simulink library "AtomicLibrary"
PostLoadFcn:
  | PacketBusGenerator
libraries: LinkLayer x5

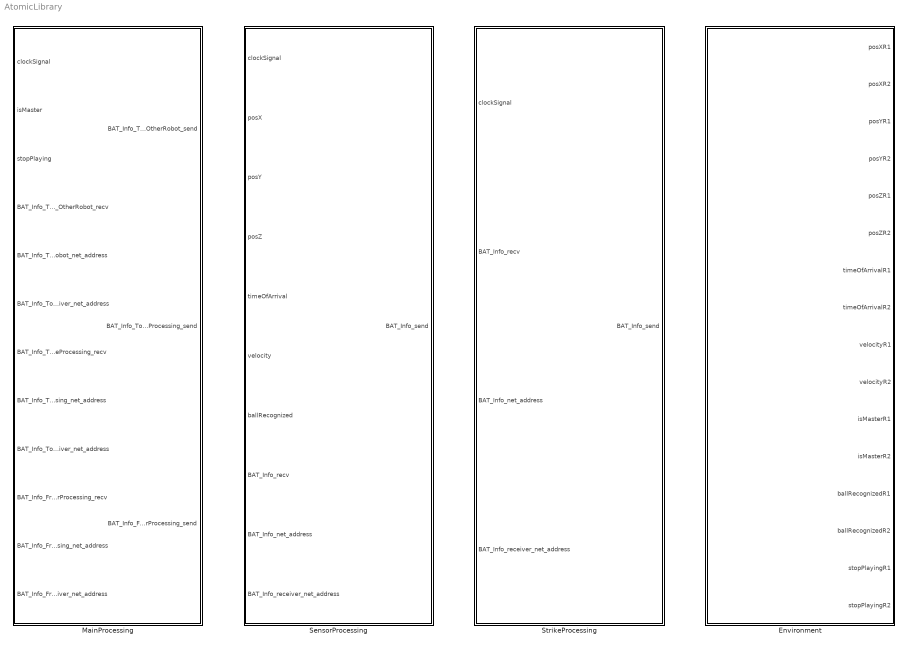
== system AtomicLibrary ==
  MainProcessing : Subsystem  Tag=id=_SXgnIKYDEeKR7Lwk7UC7tQ
  SensorProcessing : Subsystem  Tag=id=_SYKHYKYDEeKR7Lwk7UC7tQ
  StrikeProcessing : Subsystem  Tag=id=_SYeQcKYDEeKR7Lwk7UC7tQ
  Environment : Subsystem  Tag=id=_SY2q8KYDEeKR7Lwk7UC7tQ

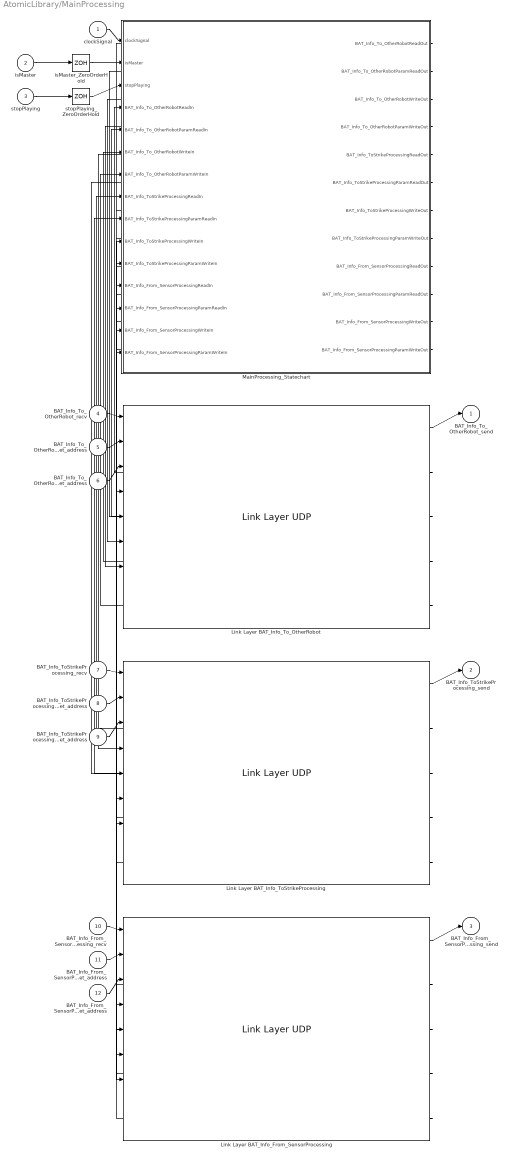
== system AtomicLibrary/MainProcessing ==
  clockSignal : Inport  Tag=id=_SXupkKYDEeKR7Lwk7UC7tQ  Port=1  DataType=auto  OutDataType=fixdt(1, 16)  OutScaling=2^0  OutDataTypeStr=Inherit: auto
  isMaster : Inport  Tag=id=_SmZ-wKYDEeKR7Lwk7UC7tQ  Port=2  DataType=boolean  OutDataType=fixdt(1, 16)  OutScaling=2^0  OutDataTypeStr=boolean
  stopPlaying : Inport  Tag=id=_SnFUMKYDEeKR7Lwk7UC7tQ  Port=3  DataType=boolean  OutDataType=fixdt(1, 16)  OutScaling=2^0  OutDataTypeStr=boolean
  BAT_Info_To_OtherRobot_recv : Inport  Tag=id=_StHDsKYDEeKR7Lwk7UC7tQ  Port=4  DataType=auto  OutDataType=fixdt(1, 16)  OutScaling=2^0  UseBusObject=on  OutDataTypeStr=Inherit: auto
      settings: BusObject=PacketBus
  BAT_Info_To_OtherRobot_net_address : Inport  Tag=id=_StIR0aYDEeKR7Lwk7UC7tQ  Port=5  DataType=uint8  OutDataType=fixdt(1, 16)  OutScaling=2^0  OutDataTypeStr=uint8
  BAT_Info_To_OtherRobot_receiver_net_address : Inport  Tag=id=_StI44KYDEeKR7Lwk7UC7tQ  Port=6  DataType=uint8  OutDataType=fixdt(1, 16)  OutScaling=2^0  OutDataTypeStr=uint8
  BAT_Info_ToStrikeProcessing_recv : Inport  Tag=id=_St01YKYDEeKR7Lwk7UC7tQ  Port=7  DataType=auto  OutDataType=fixdt(1, 16)  OutScaling=2^0  UseBusObject=on  OutDataTypeStr=Inherit: auto
      settings: BusObject=PacketBus
  BAT_Info_ToStrikeProcessing_net_address : Inport  Tag=id=_St3RoKYDEeKR7Lwk7UC7tQ  Port=8  DataType=uint8  OutDataType=fixdt(1, 16)  OutScaling=2^0  OutDataTypeStr=uint8
  BAT_Info_ToStrikeProcessing_receiver_net_address : Inport  Tag=id=_St34sKYDEeKR7Lwk7UC7tQ  Port=9  DataType=uint8  OutDataType=fixdt(1, 16)  OutScaling=2^0  OutDataTypeStr=uint8
  BAT_Info_From_SensorProcessing_recv : Inport  Tag=id=_SujOIKYDEeKR7Lwk7UC7tQ  Port=10  DataType=auto  OutDataType=fixdt(1, 16)  OutScaling=2^0  UseBusObject=on  OutDataTypeStr=Inherit: auto
      settings: BusObject=PacketBus
  BAT_Info_From_SensorProcessing_net_address : Inport  Tag=id=_SulqYKYDEeKR7Lwk7UC7tQ  Port=11  DataType=uint8  OutDataType=fixdt(1, 16)  OutScaling=2^0  OutDataTypeStr=uint8
  BAT_Info_From_SensorProcessing_receiver_net_address : Inport  Tag=id=_SunfkKYDEeKR7Lwk7UC7tQ  Port=12  DataType=uint8  OutDataType=fixdt(1, 16)  OutScaling=2^0  OutDataTypeStr=uint8
  BAT_Info_To_OtherRobot_send : Outport  Tag=id=_StGcoKYDEeKR7Lwk7UC7tQ  Port=1  DataType=auto  OutDataType=fixdt(1, 16)  OutScaling=2^0  UseBusObject=on  OutDataTypeStr=Inherit: auto
      settings: BusObject=PacketBus
  BAT_Info_ToStrikeProcessing_send : Outport  Tag=id=_St0OUKYDEeKR7Lwk7UC7tQ  Port=2  DataType=auto  OutDataType=fixdt(1, 16)  OutScaling=2^0  UseBusObject=on  OutDataTypeStr=Inherit: auto
      settings: BusObject=PacketBus
  BAT_Info_From_SensorProcessing_send : Outport  Tag=id=_SuinEKYDEeKR7Lwk7UC7tQ  Port=3  DataType=auto  OutDataType=fixdt(1, 16)  OutScaling=2^0  UseBusObject=on  OutDataTypeStr=Inherit: auto
      settings: BusObject=PacketBus
  MainProcessing_Statechart : Stateflow chart  Tag=id=_SXeK4KYDEeKR7Lwk7UC7tQ
  isMaster_ZeroOrderHold : ZeroOrderHold  Tag=id=_Smk94KYDEeKR7Lwk7UC7tQ  SampleTime=10.0
  stopPlaying_ZeroOrderHold : ZeroOrderHold  Tag=id=_SnJloKYDEeKR7Lwk7UC7tQ  SampleTime=10.0
  Link Layer BAT_Info_To_OtherRobot : LinkLayer/Link Layer UDP  DelayMin=2  DelayMax=100  MessageLossProbability=0
  Link Layer BAT_Info_ToStrikeProcessing : LinkLayer/Link Layer UDP  DelayMin=2  DelayMax=100  MessageLossProbability=0
  Link Layer BAT_Info_From_SensorProcessing : LinkLayer/Link Layer UDP  DelayMin=2  DelayMax=100  MessageLossProbability=0
  wires:
  clockSignal/1 -> MainProcessing_Statechart/1(clockSignal)
  isMaster/1 -> isMaster_ZeroOrderHold/1
  isMaster_ZeroOrderHold/1 -> MainProcessing_Statechart/2(isMaster)
  stopPlaying/1 -> stopPlaying_ZeroOrderHold/1
  stopPlaying_ZeroOrderHold/1 -> MainProcessing_Statechart/3(stopPlaying)
  Link Layer BAT_Info_To_OtherRobot/1 -> BAT_Info_To_OtherRobot_send/1
  BAT_Info_To_OtherRobot_recv/1 -> Link Layer BAT_Info_To_OtherRobot/1
  MainProcessing_Statechart/1(BAT_Info_To_OtherRobotReadOut) -> Link Layer BAT_Info_To_OtherRobot/4
  Link Layer BAT_Info_To_OtherRobot/2 -> MainProcessing_Statechart/4(BAT_Info_To_OtherRobotReadIn)
  Link Layer BAT_Info_To_OtherRobot/3 -> MainProcessing_Statechart/5(BAT_Info_To_OtherRobotParamReadIn)
  MainProcessing_Statechart/2(BAT_Info_To_OtherRobotParamReadOut) -> Link Layer BAT_Info_To_OtherRobot/5
  MainProcessing_Statechart/3(BAT_Info_To_OtherRobotWriteOut) -> Link Layer BAT_Info_To_OtherRobot/6
  MainProcessing_Statechart/4(BAT_Info_To_OtherRobotParamWriteOut) -> Link Layer BAT_Info_To_OtherRobot/7
  Link Layer BAT_Info_To_OtherRobot/4 -> MainProcessing_Statechart/6(BAT_Info_To_OtherRobotWriteIn)
  Link Layer BAT_Info_To_OtherRobot/5 -> MainProcessing_Statechart/7(BAT_Info_To_OtherRobotParamWriteIn)
  BAT_Info_To_OtherRobot_net_address/1 -> Link Layer BAT_Info_To_OtherRobot/2
  BAT_Info_To_OtherRobot_receiver_net_address/1 -> Link Layer BAT_Info_To_OtherRobot/3
  Link Layer BAT_Info_ToStrikeProcessing/1 -> BAT_Info_ToStrikeProcessing_send/1
  BAT_Info_ToStrikeProcessing_recv/1 -> Link Layer BAT_Info_ToStrikeProcessing/1
  MainProcessing_Statechart/5(BAT_Info_ToStrikeProcessingReadOut) -> Link Layer BAT_Info_ToStrikeProcessing/4
  Link Layer BAT_Info_ToStrikeProcessing/2 -> MainProcessing_Statechart/8(BAT_Info_ToStrikeProcessingReadIn)
  Link Layer BAT_Info_ToStrikeProcessing/3 -> MainProcessing_Statechart/9(BAT_Info_ToStrikeProcessingParamReadIn)
  MainProcessing_Statechart/6(BAT_Info_ToStrikeProcessingParamReadOut) -> Link Layer BAT_Info_ToStrikeProcessing/5
  MainProcessing_Statechart/7(BAT_Info_ToStrikeProcessingWriteOut) -> Link Layer BAT_Info_ToStrikeProcessing/6
  MainProcessing_Statechart/8(BAT_Info_ToStrikeProcessingParamWriteOut) -> Link Layer BAT_Info_ToStrikeProcessing/7
  Link Layer BAT_Info_ToStrikeProcessing/4 -> MainProcessing_Statechart/10(BAT_Info_ToStrikeProcessingWriteIn)
  Link Layer BAT_Info_ToStrikeProcessing/5 -> MainProcessing_Statechart/11(BAT_Info_ToStrikeProcessingParamWriteIn)
  BAT_Info_ToStrikeProcessing_net_address/1 -> Link Layer BAT_Info_ToStrikeProcessing/2
  BAT_Info_ToStrikeProcessing_receiver_net_address/1 -> Link Layer BAT_Info_ToStrikeProcessing/3
  Link Layer BAT_Info_From_SensorProcessing/1 -> BAT_Info_From_SensorProcessing_send/1
  BAT_Info_From_SensorProcessing_recv/1 -> Link Layer BAT_Info_From_SensorProcessing/1
  MainProcessing_Statechart/9(BAT_Info_From_SensorProcessingReadOut) -> Link Layer BAT_Info_From_SensorProcessing/4
  Link Layer BAT_Info_From_SensorProcessing/2 -> MainProcessing_Statechart/12(BAT_Info_From_SensorProcessingReadIn)
  Link Layer BAT_Info_From_SensorProcessing/3 -> MainProcessing_Statechart/13(BAT_Info_From_SensorProcessingParamReadIn)
  MainProcessing_Statechart/10(BAT_Info_From_SensorProcessingParamReadOut) -> Link Layer BAT_Info_From_SensorProcessing/5
  MainProcessing_Statechart/11(BAT_Info_From_SensorProcessingWriteOut) -> Link Layer BAT_Info_From_SensorProcessing/6
  MainProcessing_Statechart/12(BAT_Info_From_SensorProcessingParamWriteOut) -> Link Layer BAT_Info_From_SensorProcessing/7
  Link Layer BAT_Info_From_SensorProcessing/4 -> MainProcessing_Statechart/14(BAT_Info_From_SensorProcessingWriteIn)
  Link Layer BAT_Info_From_SensorProcessing/5 -> MainProcessing_Statechart/15(BAT_Info_From_SensorProcessingParamWriteIn)
  BAT_Info_From_SensorProcessing_net_address/1 -> Link Layer BAT_Info_From_SensorProcessing/2
  BAT_Info_From_SensorProcessing_receiver_net_address/1 -> Link Layer BAT_Info_From_SensorProcessing/3

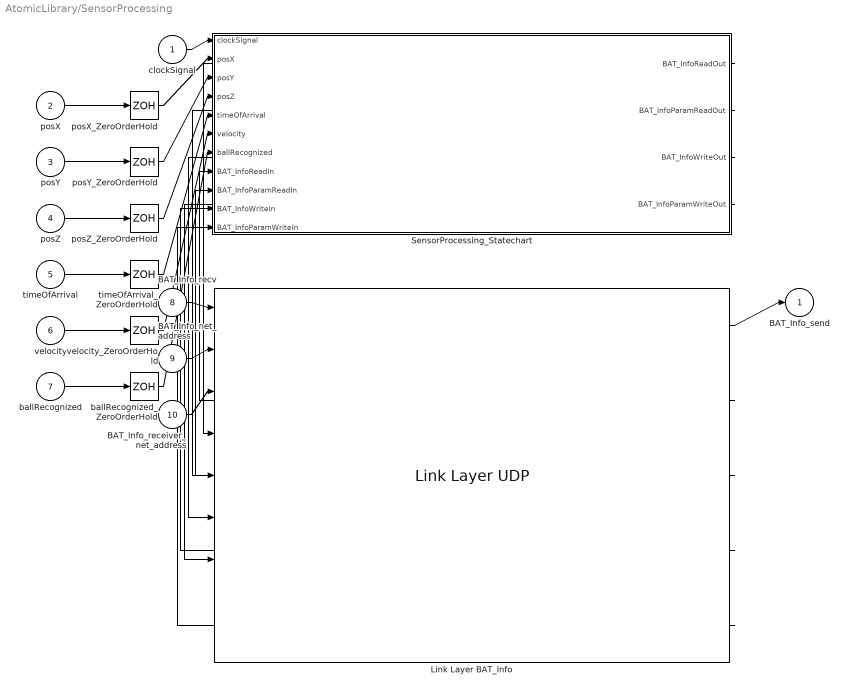
== system AtomicLibrary/SensorProcessing ==
  clockSignal : Inport  Tag=id=_SYLVgKYDEeKR7Lwk7UC7tQ  Port=1  DataType=auto  OutDataType=fixdt(1, 16)  OutScaling=2^0  OutDataTypeStr=Inherit: auto
  posX : Inport  Tag=id=_SnjOQKYDEeKR7Lwk7UC7tQ  Port=2  DataType=double  OutDataType=fixdt(1, 16)  OutScaling=2^0  OutDataTypeStr=double
  posY : Inport  Tag=id=_SoH2AKYDEeKR7Lwk7UC7tQ  Port=3  DataType=double  OutDataType=fixdt(1, 16)  OutScaling=2^0  OutDataTypeStr=double
  posZ : Inport  Tag=id=_SoozYKYDEeKR7Lwk7UC7tQ  Port=4  DataType=double  OutDataType=fixdt(1, 16)  OutScaling=2^0  OutDataTypeStr=double
  timeOfArrival : Inport  Tag=id=_SpS6sKYDEeKR7Lwk7UC7tQ  Port=5  DataType=double  OutDataType=fixdt(1, 16)  OutScaling=2^0  OutDataTypeStr=double
  velocity : Inport  Tag=id=_Sp5XoKYDEeKR7Lwk7UC7tQ  Port=6  DataType=double  OutDataType=fixdt(1, 16)  OutScaling=2^0  OutDataTypeStr=double
  ballRecognized : Inport  Tag=id=_SqplkKYDEeKR7Lwk7UC7tQ  Port=7  DataType=boolean  OutDataType=fixdt(1, 16)  OutScaling=2^0  OutDataTypeStr=boolean
  BAT_Info_recv : Inport  Tag=id=_SvNVcKYDEeKR7Lwk7UC7tQ  Port=8  DataType=auto  OutDataType=fixdt(1, 16)  OutScaling=2^0  UseBusObject=on  OutDataTypeStr=Inherit: auto
      settings: BusObject=PacketBus
  BAT_Info_net_address : Inport  Tag=id=_SvPKoKYDEeKR7Lwk7UC7tQ  Port=9  DataType=uint8  OutDataType=fixdt(1, 16)  OutScaling=2^0  OutDataTypeStr=uint8
  BAT_Info_receiver_net_address : Inport  Tag=id=_SvPxsKYDEeKR7Lwk7UC7tQ  Port=10  DataType=uint8  OutDataType=fixdt(1, 16)  OutScaling=2^0  OutDataTypeStr=uint8
  BAT_Info_send : Outport  Tag=id=_SvMuYKYDEeKR7Lwk7UC7tQ  Port=1  DataType=auto  OutDataType=fixdt(1, 16)  OutScaling=2^0  UseBusObject=on  OutDataTypeStr=Inherit: auto
      settings: BusObject=PacketBus
  SensorProcessing_Statechart : Stateflow chart  Tag=id=_SYI5QKYDEeKR7Lwk7UC7tQ
  posX_ZeroOrderHold : ZeroOrderHold  Tag=id=_Snm4oKYDEeKR7Lwk7UC7tQ  SampleTime=10.0
  posY_ZeroOrderHold : ZeroOrderHold  Tag=id=_SoK5UKYDEeKR7Lwk7UC7tQ  SampleTime=10.0
  posZ_ZeroOrderHold : ZeroOrderHold  Tag=id=_Sotr4KYDEeKR7Lwk7UC7tQ  SampleTime=10.0
  timeOfArrival_ZeroOrderHold : ZeroOrderHold  Tag=id=_SpXMIKYDEeKR7Lwk7UC7tQ  SampleTime=10.0
  velocity_ZeroOrderHold : ZeroOrderHold  Tag=id=_Sp_eQKYDEeKR7Lwk7UC7tQ  SampleTime=10.0
  ballRecognized_ZeroOrderHold : ZeroOrderHold  Tag=id=_SqtP8KYDEeKR7Lwk7UC7tQ  SampleTime=10.0
  Link Layer BAT_Info : LinkLayer/Link Layer UDP  DelayMin=2  DelayMax=100  MessageLossProbability=0
  wires:
  clockSignal/1 -> SensorProcessing_Statechart/1(clockSignal)
  posX/1 -> posX_ZeroOrderHold/1
  posX_ZeroOrderHold/1 -> SensorProcessing_Statechart/2(posX)
  posY/1 -> posY_ZeroOrderHold/1
  posY_ZeroOrderHold/1 -> SensorProcessing_Statechart/3(posY)
  posZ/1 -> posZ_ZeroOrderHold/1
  posZ_ZeroOrderHold/1 -> SensorProcessing_Statechart/4(posZ)
  timeOfArrival/1 -> timeOfArrival_ZeroOrderHold/1
  timeOfArrival_ZeroOrderHold/1 -> SensorProcessing_Statechart/5(timeOfArrival)
  velocity/1 -> velocity_ZeroOrderHold/1
  velocity_ZeroOrderHold/1 -> SensorProcessing_Statechart/6(velocity)
  ballRecognized/1 -> ballRecognized_ZeroOrderHold/1
  ballRecognized_ZeroOrderHold/1 -> SensorProcessing_Statechart/7(ballRecognized)
  Link Layer BAT_Info/1 -> BAT_Info_send/1
  BAT_Info_recv/1 -> Link Layer BAT_Info/1
  SensorProcessing_Statechart/1(BAT_InfoReadOut) -> Link Layer BAT_Info/4
  Link Layer BAT_Info/2 -> SensorProcessing_Statechart/8(BAT_InfoReadIn)
  Link Layer BAT_Info/3 -> SensorProcessing_Statechart/9(BAT_InfoParamReadIn)
  SensorProcessing_Statechart/2(BAT_InfoParamReadOut) -> Link Layer BAT_Info/5
  SensorProcessing_Statechart/3(BAT_InfoWriteOut) -> Link Layer BAT_Info/6
  SensorProcessing_Statechart/4(BAT_InfoParamWriteOut) -> Link Layer BAT_Info/7
  Link Layer BAT_Info/4 -> SensorProcessing_Statechart/10(BAT_InfoWriteIn)
  Link Layer BAT_Info/5 -> SensorProcessing_Statechart/11(BAT_InfoParamWriteIn)
  BAT_Info_net_address/1 -> Link Layer BAT_Info/2
  BAT_Info_receiver_net_address/1 -> Link Layer BAT_Info/3

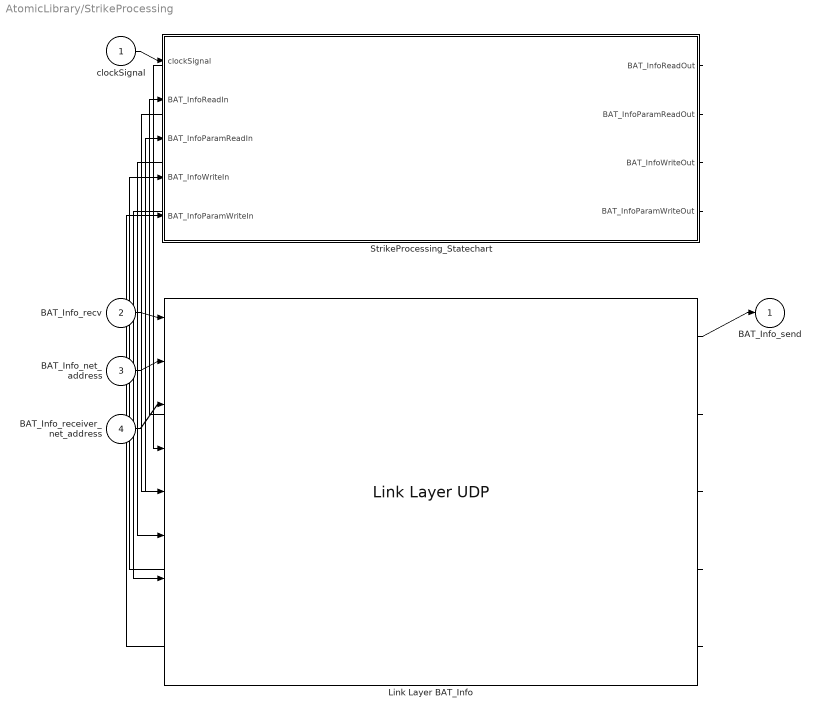
== system AtomicLibrary/StrikeProcessing ==
  clockSignal : Inport  Tag=id=_SYgFoKYDEeKR7Lwk7UC7tQ  Port=1  DataType=auto  OutDataType=fixdt(1, 16)  OutScaling=2^0  OutDataTypeStr=Inherit: auto
  BAT_Info_recv : Inport  Tag=id=_SsIMQKYDEeKR7Lwk7UC7tQ  Port=2  DataType=auto  OutDataType=fixdt(1, 16)  OutScaling=2^0  UseBusObject=on  OutDataTypeStr=Inherit: auto
      settings: BusObject=PacketBus
  BAT_Info_net_address : Inport  Tag=id=_SsYD4KYDEeKR7Lwk7UC7tQ  Port=3  DataType=uint8  OutDataType=fixdt(1, 16)  OutScaling=2^0  OutDataTypeStr=uint8
  BAT_Info_receiver_net_address : Inport  Tag=id=_SsZSAKYDEeKR7Lwk7UC7tQ  Port=4  DataType=uint8  OutDataType=fixdt(1, 16)  OutScaling=2^0  OutDataTypeStr=uint8
  BAT_Info_send : Outport  Tag=id=_SsG-IKYDEeKR7Lwk7UC7tQ  Port=1  DataType=auto  OutDataType=fixdt(1, 16)  OutScaling=2^0  UseBusObject=on  OutDataTypeStr=Inherit: auto
      settings: BusObject=PacketBus
  StrikeProcessing_Statechart : Stateflow chart  Tag=id=_SYbNIKYDEeKR7Lwk7UC7tQ
  Link Layer BAT_Info : LinkLayer/Link Layer UDP  DelayMin=2  DelayMax=100  MessageLossProbability=0
  wires:
  clockSignal/1 -> StrikeProcessing_Statechart/1(clockSignal)
  Link Layer BAT_Info/1 -> BAT_Info_send/1
  BAT_Info_recv/1 -> Link Layer BAT_Info/1
  StrikeProcessing_Statechart/1(BAT_InfoReadOut) -> Link Layer BAT_Info/4
  Link Layer BAT_Info/2 -> StrikeProcessing_Statechart/2(BAT_InfoReadIn)
  Link Layer BAT_Info/3 -> StrikeProcessing_Statechart/3(BAT_InfoParamReadIn)
  StrikeProcessing_Statechart/2(BAT_InfoParamReadOut) -> Link Layer BAT_Info/5
  StrikeProcessing_Statechart/3(BAT_InfoWriteOut) -> Link Layer BAT_Info/6
  StrikeProcessing_Statechart/4(BAT_InfoParamWriteOut) -> Link Layer BAT_Info/7
  Link Layer BAT_Info/4 -> StrikeProcessing_Statechart/4(BAT_InfoWriteIn)
  Link Layer BAT_Info/5 -> StrikeProcessing_Statechart/5(BAT_InfoParamWriteIn)
  BAT_Info_net_address/1 -> Link Layer BAT_Info/2
  BAT_Info_receiver_net_address/1 -> Link Layer BAT_Info/3

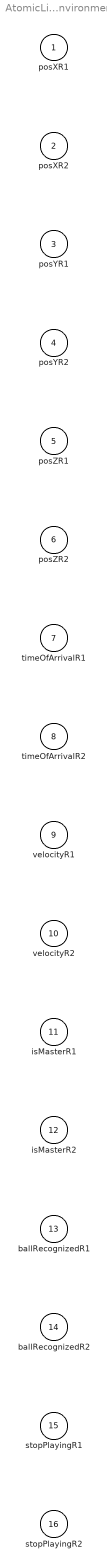
== system AtomicLibrary/Environment ==
  posXR1 : Outport  Tag=id=_SfmMIKYDEeKR7Lwk7UC7tQ  Port=1  DataType=double  OutDataType=fixdt(1, 16)  OutScaling=2^0  OutDataTypeStr=double
  posXR2 : Outport  Tag=id=_SgUk4KYDEeKR7Lwk7UC7tQ  Port=2  DataType=double  OutDataType=fixdt(1, 16)  OutScaling=2^0  OutDataTypeStr=double
  posYR1 : Outport  Tag=id=_Sg3-gKYDEeKR7Lwk7UC7tQ  Port=3  DataType=double  OutDataType=fixdt(1, 16)  OutScaling=2^0  OutDataTypeStr=double
  posYR2 : Outport  Tag=id=_Shr20KYDEeKR7Lwk7UC7tQ  Port=4  DataType=double  OutDataType=fixdt(1, 16)  OutScaling=2^0  OutDataTypeStr=double
  posZR1 : Outport  Tag=id=_Sh-xwKYDEeKR7Lwk7UC7tQ  Port=5  DataType=double  OutDataType=fixdt(1, 16)  OutScaling=2^0  OutDataTypeStr=double
  posZR2 : Outport  Tag=id=_SiMNIKYDEeKR7Lwk7UC7tQ  Port=6  DataType=double  OutDataType=fixdt(1, 16)  OutScaling=2^0  OutDataTypeStr=double
  timeOfArrivalR1 : Outport  Tag=id=_Sia2oKYDEeKR7Lwk7UC7tQ  Port=7  DataType=double  OutDataType=fixdt(1, 16)  OutScaling=2^0  OutDataTypeStr=double
  timeOfArrivalR2 : Outport  Tag=id=_SitKgKYDEeKR7Lwk7UC7tQ  Port=8  DataType=double  OutDataType=fixdt(1, 16)  OutScaling=2^0  OutDataTypeStr=double
  velocityR1 : Outport  Tag=id=_SjBTkKYDEeKR7Lwk7UC7tQ  Port=9  DataType=double  OutDataType=fixdt(1, 16)  OutScaling=2^0  OutDataTypeStr=double
  velocityR2 : Outport  Tag=id=_SjP9EKYDEeKR7Lwk7UC7tQ  Port=10  DataType=double  OutDataType=fixdt(1, 16)  OutScaling=2^0  OutDataTypeStr=double
  isMasterR1 : Outport  Tag=id=_SjgbwKYDEeKR7Lwk7UC7tQ  Port=11  DataType=boolean  OutDataType=fixdt(1, 16)  OutScaling=2^0  OutDataTypeStr=boolean
  isMasterR2 : Outport  Tag=id=_SjtQEKYDEeKR7Lwk7UC7tQ  Port=12  DataType=boolean  OutDataType=fixdt(1, 16)  OutScaling=2^0  OutDataTypeStr=boolean
  ballRecognizedR1 : Outport  Tag=id=_Sj-84KYDEeKR7Lwk7UC7tQ  Port=13  DataType=boolean  OutDataType=fixdt(1, 16)  OutScaling=2^0  OutDataTypeStr=boolean
  ballRecognizedR2 : Outport  Tag=id=_SkRQwKYDEeKR7Lwk7UC7tQ  Port=14  DataType=boolean  OutDataType=fixdt(1, 16)  OutScaling=2^0  OutDataTypeStr=boolean
  stopPlayingR1 : Outport  Tag=id=_Sky1MKYDEeKR7Lwk7UC7tQ  Port=15  DataType=boolean  OutDataType=fixdt(1, 16)  OutScaling=2^0  OutDataTypeStr=boolean
  stopPlayingR2 : Outport  Tag=id=_SlXc8KYDEeKR7Lwk7UC7tQ  Port=16  DataType=boolean  OutDataType=fixdt(1, 16)  OutScaling=2^0  OutDataTypeStr=boolean

== stateflow chart MainProcessing/MainProcessing_Statechart ==
  state chart
    state chartRegion [parallel]
      settings: executionOrder=2
      state init
        state MainProcessingPort_BAT_Info_To_Other_Robot [parallel]
          settings: executionOrder=3
          state Init
          state YourTurn
            entry: c0=reset();
          state MyTurn
            entry: c0=reset();
          state Timeout
          state Inv_Error
          Init -> YourTurn [order 2] : [isMaster == true && BAT_Info_ReceivedBySP == true]
              | {[BAT_Info_To_OtherRobotWriteOut, BAT_Info_To_OtherRobotParamWriteOut] = BAT_Info_To_OtherRobot_enqueue(EVT_TURN_POSX, BAT_Info_To_OtherRobotWriteOut, double(posXReceivedBySP), BAT_Info_To_OtherRobotParamWriteOut)
              | [BAT_Info_To_OtherRobotWriteOut, BAT_Info_To_OtherRobotParamWriteOut] = BAT_Info_To_OtherRobot_enqueue(EVT_TURN_POSY, BAT_Info_To_OtherRobotWriteOut, double(posYReceivedBySP), BAT_Info_To_OtherRobotParamWriteOut)
              | [BAT_Info_To_OtherRobotWriteOut, BAT_Info_To_OtherRobotParamWriteOut] = BAT_Info_To_OtherRobot_enqueue(EVT_TURN_POSZ, BAT_Info_To_OtherRobotWriteOut, double(posZReceivedBySP), BAT_Info_To_OtherRobotParamWriteOut)
              | [BAT_Info_To_OtherRobotWriteOut, BAT_Info_To_OtherRobotParamWriteOut] = BAT_Info_To_OtherRobot_enqueue(EVT_TURN_TIMEOFARRIVAL, BAT_Info_To_OtherRobotWriteOut, double(timeOfArrivalReceivedBySP), BAT_Info_To_OtherRobotParamWriteOut)
              | [BAT_Info_To_OtherRobotWriteOut, BAT_Info_To_OtherRobotParamWriteOut] = BAT_Info_To_OtherRobot_enqueue(EVT_TURN_VELOCITY, BAT_Info_To_OtherRobotWriteOut, double(velocityReceivedBySP), BAT_Info_To_OtherRobotParamWriteOut)
              | ; BAT_Info_ReceivedBySP = false ; }
          YourTurn -> Init [order 1] : [BAT_Info_To_OtherRobot_checkQueue(EVT_STOPPLAYING, BAT_Info_To_OtherRobotReadOut)]
              | {[BAT_Info_To_OtherRobotReadOut, BAT_Info_To_OtherRobotParamReadOut] = BAT_Info_To_OtherRobot_dequeue(EVT_STOPPLAYING, BAT_Info_To_OtherRobotReadOut, BAT_Info_To_OtherRobotParamReadOut); }
          MyTurn -> Init [order 1] : [stopPlaying == true]
              | {[BAT_Info_To_OtherRobotWriteOut, BAT_Info_To_OtherRobotParamWriteOut] = BAT_Info_To_OtherRobot_enqueue(EVT_STOPPLAYING, BAT_Info_To_OtherRobotWriteOut, 0, BAT_Info_To_OtherRobotParamWriteOut); }
          Timeout -> Init
          Init -> MyTurn [order 1] : [BAT_Info_To_OtherRobot_checkQueue(EVT_TURN_POSX, BAT_Info_To_OtherRobotReadOut) && BAT_Info_To_OtherRobot_checkQueue(EVT_TURN_POSY, BAT_Info_To_OtherRobotReadOut) && BAT_Info_To_OtherRobot_checkQueue(EVT_TURN_POSZ, BAT_Info_To_OtherRobotReadOut) && BAT_Info_To_OtherRobot_checkQueue(EVT_TURN_TIMEOFARRIVAL, BAT_Info_To_OtherRobotReadOut) && BAT_Info_To_OtherRobot_checkQueue(EVT_TURN_VELOCITY, BAT_Info_To_OtherRobotReadOut)]
              | {[BAT_Info_To_OtherRobotReadOut, BAT_Info_To_OtherRobotParamReadOut, tmp_var_1] = BAT_Info_To_OtherRobot_dequeue(EVT_TURN_POSX, BAT_Info_To_OtherRobotReadOut, BAT_Info_To_OtherRobotParamReadOut);
              | [BAT_Info_To_OtherRobotReadOut, BAT_Info_To_OtherRobotParamReadOut, tmp_var_2] = BAT_Info_To_OtherRobot_dequeue(EVT_TURN_POSY, BAT_Info_To_OtherRobotReadOut, BAT_Info_To_OtherRobotParamReadOut);
              | [BAT_Info_To_OtherRobotReadOut, BAT_Info_To_OtherRobotParamReadOut, tmp_var_3] = BAT_Info_To_OtherRobot_dequeue(EVT_TURN_POSZ, BAT_Info_To_OtherRobotReadOut, BAT_Info_To_OtherRobotParamReadOut);
              | [BAT_Info_To_OtherRobotReadOut, BAT_Info_To_OtherRobotParamReadOut, tmp_var_4] = BAT_Info_To_OtherRobot_dequeue(EVT_TURN_TIMEOFARRIVAL, BAT_Info_To_OtherRobotReadOut, BAT_Info_To_OtherRobotParamReadOut);
              | [BAT_Info_To_OtherRobotReadOut, BAT_Info_To_OtherRobotParamReadOut, tmp_var_5] = BAT_Info_To_OtherRobot_dequeue(EVT_TURN_VELOCITY, BAT_Info_To_OtherRobotReadOut, BAT_Info_To_OtherRobotParamReadOut); posXReceivedByRobot = tmp_var_1 ;  posYReceivedByRobot = tmp_var_2 ;  posZReceivedByRobot = tmp_var_3 ;  timeOfArrivalReceivedByRobot = tmp_var_4 ;  velocityReceivedByRobot = tmp_var_5 ;  BAT_Info_ReceivedByRobot = true ; }
          MyTurn -> YourTurn [order 3] : [BAT_Info_ReceivedBySP == true]
              | {[BAT_Info_To_OtherRobotWriteOut, BAT_Info_To_OtherRobotParamWriteOut] = BAT_Info_To_OtherRobot_enqueue(EVT_TURN_POSX, BAT_Info_To_OtherRobotWriteOut, double(posXReceivedByRobot), BAT_Info_To_OtherRobotParamWriteOut)
              | [BAT_Info_To_OtherRobotWriteOut, BAT_Info_To_OtherRobotParamWriteOut] = BAT_Info_To_OtherRobot_enqueue(EVT_TURN_POSY, BAT_Info_To_OtherRobotWriteOut, double(posYReceivedBySP), BAT_Info_To_OtherRobotParamWriteOut)
              | [BAT_Info_To_OtherRobotWriteOut, BAT_Info_To_OtherRobotParamWriteOut] = BAT_Info_To_OtherRobot_enqueue(EVT_TURN_POSZ, BAT_Info_To_OtherRobotWriteOut, double(posZReceivedBySP), BAT_Info_To_OtherRobotParamWriteOut)
              | [BAT_Info_To_OtherRobotWriteOut, BAT_Info_To_OtherRobotParamWriteOut] = BAT_Info_To_OtherRobot_enqueue(EVT_TURN_TIMEOFARRIVAL, BAT_Info_To_OtherRobotWriteOut, double(timeOfArrivalReceivedBySP), BAT_Info_To_OtherRobotParamWriteOut)
              | [BAT_Info_To_OtherRobotWriteOut, BAT_Info_To_OtherRobotParamWriteOut] = BAT_Info_To_OtherRobot_enqueue(EVT_TURN_VELOCITY, BAT_Info_To_OtherRobotWriteOut, double(velocityReceivedBySP), BAT_Info_To_OtherRobotParamWriteOut)
              | ; BAT_Info_ReceivedBySP = false ; }
          YourTurn -> MyTurn [order 3] : [BAT_Info_To_OtherRobot_checkQueue(EVT_TURN_POSX, BAT_Info_To_OtherRobotReadOut) && BAT_Info_To_OtherRobot_checkQueue(EVT_TURN_POSY, BAT_Info_To_OtherRobotReadOut) && BAT_Info_To_OtherRobot_checkQueue(EVT_TURN_POSZ, BAT_Info_To_OtherRobotReadOut) && BAT_Info_To_OtherRobot_checkQueue(EVT_TURN_TIMEOFARRIVAL, BAT_Info_To_OtherRobotReadOut) && BAT_Info_To_OtherRobot_checkQueue(EVT_TURN_VELOCITY, BAT_Info_To_OtherRobotReadOut)]
              | {[BAT_Info_To_OtherRobotReadOut, BAT_Info_To_OtherRobotParamReadOut, tmp_var_1] = BAT_Info_To_OtherRobot_dequeue(EVT_TURN_POSX, BAT_Info_To_OtherRobotReadOut, BAT_Info_To_OtherRobotParamReadOut);
              | [BAT_Info_To_OtherRobotReadOut, BAT_Info_To_OtherRobotParamReadOut, tmp_var_2] = BAT_Info_To_OtherRobot_dequeue(EVT_TURN_POSY, BAT_Info_To_OtherRobotReadOut, BAT_Info_To_OtherRobotParamReadOut);
              | [BAT_Info_To_OtherRobotReadOut, BAT_Info_To_OtherRobotParamReadOut, tmp_var_3] = BAT_Info_To_OtherRobot_dequeue(EVT_TURN_POSZ, BAT_Info_To_OtherRobotReadOut, BAT_Info_To_OtherRobotParamReadOut);
              | [BAT_Info_To_OtherRobotReadOut, BAT_Info_To_OtherRobotParamReadOut, tmp_var_4] = BAT_Info_To_OtherRobot_dequeue(EVT_TURN_TIMEOFARRIVAL, BAT_Info_To_OtherRobotReadOut, BAT_Info_To_OtherRobotParamReadOut);
              | [BAT_Info_To_OtherRobotReadOut, BAT_Info_To_OtherRobotParamReadOut, tmp_var_5] = BAT_Info_To_OtherRobot_dequeue(EVT_TURN_VELOCITY, BAT_Info_To_OtherRobotReadOut, BAT_Info_To_OtherRobotParamReadOut); posXReceivedByRobot = tmp_var_1 ;  posYReceivedByRobot = tmp_var_2 ;  posZReceivedByRobot = tmp_var_3 ;  timeOfArrivalReceivedByRobot = tmp_var_4 ;  velocityReceivedByRobot = tmp_var_5 ;  BAT_Info_ReceivedByRobot = true ; }
          YourTurn -> Timeout [order 2] : [time(c0) >= 1.0]
          MyTurn -> Timeout [order 2] : [time(c0) >= 1.0]
          YourTurn -> Inv_Error [order 4] : [time(c0) > 1000]
          MyTurn -> Inv_Error [order 4] : [time(c0) >= 1000]
        state MainProcessingPort_BAT_Info_To_StrikeP [parallel]
          settings: executionOrder=2
          state Sending
          Sending -> Sending : [BAT_Info_ReceivedByRobot == true]
              | {[BAT_Info_ToStrikeProcessingWriteOut, BAT_Info_ToStrikeProcessingParamWriteOut] = BAT_Info_ToStrikeProcessing_enqueue(EVT_TRANSFERBATINFO_POSX, BAT_Info_ToStrikeProcessingWriteOut, double(posXReceivedByRobot), BAT_Info_ToStrikeProcessingParamWriteOut)
              | [BAT_Info_ToStrikeProcessingWriteOut, BAT_Info_ToStrikeProcessingParamWriteOut] = BAT_Info_ToStrikeProcessing_enqueue(EVT_TRANSFERBATINFO_POSY, BAT_Info_ToStrikeProcessingWriteOut, double(posYReceivedByRobot), BAT_Info_ToStrikeProcessingParamWriteOut)
              | [BAT_Info_ToStrikeProcessingWriteOut, BAT_Info_ToStrikeProcessingParamWriteOut] = BAT_Info_ToStrikeProcessing_enqueue(EVT_TRANSFERBATINFO_POSZ, BAT_Info_ToStrikeProcessingWriteOut, double(posZReceivedByRobot), BAT_Info_ToStrikeProcessingParamWriteOut)
              | [BAT_Info_ToStrikeProcessingWriteOut, BAT_Info_ToStrikeProcessingParamWriteOut] = BAT_Info_ToStrikeProcessing_enqueue(EVT_TRANSFERBATINFO_TIMEOFARRIVAL, BAT_Info_ToStrikeProcessingWriteOut, double(timeOfArrivalReceivedByRobot), BAT_Info_ToStrikeProcessingParamWriteOut)
              | [BAT_Info_ToStrikeProcessingWriteOut, BAT_Info_ToStrikeProcessingParamWriteOut] = BAT_Info_ToStrikeProcessing_enqueue(EVT_TRANSFERBATINFO_VELOCITY, BAT_Info_ToStrikeProcessingWriteOut, double(velocityReceivedByRobot), BAT_Info_ToStrikeProcessingParamWriteOut)
              | ; BAT_Info_ReceivedByRobot = false ; }
        state MainProcessingPort_BAT_Info_To_SensorP [parallel]
          settings: executionOrder=1
          state Receiving
          Receiving -> Receiving : [BAT_Info_From_SensorProcessing_checkQueue(EVT_TRANSFERBATINFO_POSX, BAT_Info_From_SensorProcessingReadOut) && BAT_Info_From_SensorProcessing_checkQueue(EVT_TRANSFERBATINFO_POSY, BAT_Info_From_SensorProcessingReadOut) && BAT_Info_From_SensorProcessing_checkQueue(EVT_TRANSFERBATINFO_POSZ, BAT_Info_From_SensorProcessingReadOut) && BAT_Info_From_SensorProcessing_checkQueue(EVT_TRANSFERBATINFO_TIMEOFARRIVAL, BAT_Info_From_SensorProcessingReadOut) && BAT_Info_From_SensorProcessing_checkQueue(EVT_TRANSFERBATINFO_VELOCITY, BAT_Info_From_SensorProcessingReadOut)]
              | {[BAT_Info_From_SensorProcessingReadOut, BAT_Info_From_SensorProcessingParamReadOut, tmp_var_1] = BAT_Info_From_SensorProcessing_dequeue(EVT_TRANSFERBATINFO_POSX, BAT_Info_From_SensorProcessingReadOut, BAT_Info_From_SensorProcessingParamReadOut);
              | [BAT_Info_From_SensorProcessingReadOut, BAT_Info_From_SensorProcessingParamReadOut, tmp_var_2] = BAT_Info_From_SensorProcessing_dequeue(EVT_TRANSFERBATINFO_POSY, BAT_Info_From_SensorProcessingReadOut, BAT_Info_From_SensorProcessingParamReadOut);
              | [BAT_Info_From_SensorProcessingReadOut, BAT_Info_From_SensorProcessingParamReadOut, tmp_var_3] = BAT_Info_From_SensorProcessing_dequeue(EVT_TRANSFERBATINFO_POSZ, BAT_Info_From_SensorProcessingReadOut, BAT_Info_From_SensorProcessingParamReadOut);
              | [BAT_Info_From_SensorProcessingReadOut, BAT_Info_From_SensorProcessingParamReadOut, tmp_var_4] = BAT_Info_From_SensorProcessing_dequeue(EVT_TRANSFERBATINFO_TIMEOFARRIVAL, BAT_Info_From_SensorProcessingReadOut, BAT_Info_From_SensorProcessingParamReadOut);
              | [BAT_Info_From_SensorProcessingReadOut, BAT_Info_From_SensorProcessingParamReadOut, tmp_var_5] = BAT_Info_From_SensorProcessing_dequeue(EVT_TRANSFERBATINFO_VELOCITY, BAT_Info_From_SensorProcessingReadOut, BAT_Info_From_SensorProcessingParamReadOut); posXReceivedBySP = tmp_var_1 ;  posYReceivedBySP = tmp_var_2 ;  posZReceivedBySP = tmp_var_3 ;  timeOfArrivalReceivedBySP = tmp_var_4 ;  velocityReceivedBySP = tmp_var_5 ;  BAT_Info_ReceivedBySP = true ; }
    state DataInit [parallel]
      settings: executionOrder=1
    DataInit -> DataInit : {BAT_Info_To_OtherRobotWriteOut = BAT_Info_To_OtherRobotWriteIn;
        | BAT_Info_To_OtherRobotParamWriteOut = BAT_Info_To_OtherRobotParamWriteIn;
        | BAT_Info_To_OtherRobotReadOut = BAT_Info_To_OtherRobotReadIn;
        | BAT_Info_To_OtherRobotParamReadOut = BAT_Info_To_OtherRobotParamReadIn;
        | BAT_Info_ToStrikeProcessingWriteOut = BAT_Info_ToStrikeProcessingWriteIn;
        | BAT_Info_ToStrikeProcessingParamWriteOut = BAT_Info_ToStrikeProcessingParamWriteIn;
        | BAT_Info_ToStrikeProcessingReadOut = BAT_Info_ToStrikeProcessingReadIn;
        | BAT_Info_ToStrikeProcessingParamReadOut = BAT_Info_ToStrikeProcessingParamReadIn;
        | BAT_Info_From_SensorProcessingWriteOut = BAT_Info_From_SensorProcessingWriteIn;
        | BAT_Info_From_SensorProcessingParamWriteOut = BAT_Info_From_SensorProcessingParamWriteIn;
        | BAT_Info_From_SensorProcessingReadOut = BAT_Info_From_SensorProcessingReadIn;
        | BAT_Info_From_SensorProcessingParamReadOut = BAT_Info_From_SensorProcessingParamReadIn;
        | ; }
  (default) -> Init
  (default) -> Sending
  (default) -> Receiving
  (default) -> init
  (default) -> chart
  data: c0 local double =0.0; BAT_Info_ReceivedBySP local boolean; BAT_Info_ReceivedByRobot local boolean; posXReceivedBySP local double; posXReceivedByRobot local double; posYReceivedBySP local double; posYReceivedByRobot local double; posZReceivedBySP local double; posZReceivedByRobot local double; timeOfArrivalReceivedBySP local double; timeOfArrivalReceivedByRobot local double; velocityReceivedBySP local double; velocityReceivedByRobot local double; clock function_input double; logicalTime function_output uint32; clock function_output double; event function_input uint8; evtQueueIn function_input uint8 size=[10,2]; param function_input double; paramQueueIn function_input double size=[10]; evtQueue function_output uint8 size=[10,2]; paramQueue function_output double size=[10]; event function_input uint8; evtQueueIn function_input uint8 size=[10,2]; paramQueueIn function_input double size=[10]; evtQueue function_output uint8 size=[10,2]; paramQueue function_output double size=[10]; parameter function_output double; event function_input uint8; evtQueue function_input uint8 size=[10,2]; available function_output boolean; event function_input uint8; evtQueueIn function_input uint8 size=[10,2]; param function_input double; paramQueueIn function_input double size=[10]; evtQueue function_output uint8 size=[10,2]; paramQueue function_output double size=[10]; event function_input uint8; evtQueueIn function_input uint8 size=[10,2]; paramQueueIn function_input double size=[10]; evtQueue function_output uint8 size=[10,2]; paramQueue function_output double size=[10]; parameter function_output double; event function_input uint8; evtQueue function_input uint8 size=[10,2]; available function_output boolean; event function_input uint8; evtQueueIn function_input uint8 size=[10,2]; param function_input double; paramQueueIn function_input double size=[10]; evtQueue function_output uint8 size=[10,2]; paramQueue function_output double size=[10]; event function_input uint8; evtQueueIn function_input uint8 size=[10,2]; paramQueueIn function_input double size=[10]; evtQueue function_output uint8 size=[10,2]; paramQueue function_output double size=[10]; parameter function_output double; event function_input uint8; evtQueue function_input uint8 size=[10,2]; available function_output boolean; clockSignal input double; isMaster input boolean; stopPlaying input boolean; BAT_Info_To_OtherRobotReadIn input uint8 size=[10,2]; BAT_Info_To_OtherRobotParamReadIn input double size=10; BAT_Info_To_OtherRobotWriteIn input uint8 size=[10,2]; BAT_Info_To_OtherRobotParamWriteIn input double size=10; BAT_Info_ToStrikeProcessingReadIn input uint8 size=[10,2]; BAT_Info_ToStrikeProcessingParamReadIn input double size=10; BAT_Info_ToStrikeProcessingWriteIn input uint8 size=[10,2]; BAT_Info_ToStrikeProcessingParamWriteIn input double size=10; BAT_Info_From_SensorProcessingReadIn input uint8 size=[10,2]; BAT_Info_From_SensorProcessingParamReadIn input double size=10; BAT_Info_From_SensorProcessingWriteIn input uint8 size=[10,2]; BAT_Info_From_SensorProcessingParamWriteIn input double size=10; BAT_Info_To_OtherRobotReadOut output uint8 size=[10,2]; BAT_Info_To_OtherRobotParamReadOut output double size=10; BAT_Info_To_OtherRobotWriteOut output uint8 size=[10,2]; BAT_Info_To_OtherRobotParamWriteOut output double size=10; BAT_Info_ToStrikeProcessingReadOut output uint8 size=[10,2]; BAT_Info_ToStrikeProcessingParamReadOut output double size=10; BAT_Info_ToStrikeProcessingWriteOut output uint8 size=[10,2]; BAT_Info_ToStrikeProcessingParamWriteOut output double size=10; BAT_Info_From_SensorProcessingReadOut output uint8 size=[10,2]; BAT_Info_From_SensorProcessingParamReadOut output double size=10; BAT_Info_From_SensorProcessingWriteOut output uint8 size=[10,2]; BAT_Info_From_SensorProcessingParamWriteOut output double size=10; EVT_TURN_POSX constant uint32 =1; EVT_TURN_POSY constant uint32 =2; EVT_TURN_POSZ constant uint32 =3; EVT_TURN_TIMEOFARRIVAL constant uint32 =4; EVT_TURN_VELOCITY constant uint32 =5; EVT_TRANSFERBATINFO_POSX constant uint32 =6; EVT_TRANSFERBATINFO_POSY constant uint32 =7; EVT_TRANSFERBATINFO_POSZ constant uint32 =8; EVT_TRANSFERBATINFO_TIMEOFARRIVAL constant uint32 =9; EVT_TRANSFERBATINFO_VELOCITY constant uint32 =10; EVT_STOPPLAYING constant uint32 =12; tmp_var_1 local double; tmp_var_2 local double; tmp_var_3 local double; tmp_var_4 local double; tmp_var_5 local double
  function logicalTime = time(clock):
    | function logicalTime = time(clock) 
    | 
    |  sample = 0.001;  % the sample time of the system clock 
    | 
    |  %convert to pass units of time after last reset 
    | 
    |  logicalTime = uint32((clockSignal - clock)/sample);
  function clock = reset():
    | function clock = reset() 
    | 
    |  %set clock variable to current time 
    | 
    |  clock = clockSignal;
  function [evtQueue, paramQueue] = BAT_Info_To_OtherRobot_enqueue(event, evtQueueIn, param, paramQueueIn):
    | function [evtQueue, paramQueue] = BAT_Info_To_OtherRobot_enqueue(event, evtQueueIn, param, paramQueueIn) %eml 
    |  evtQueue = evtQueueIn; 
    |  paramQueue = paramQueueIn; 
    |  for i = 1:length(evtQueue) 
    |  	if evtQueue(i) == uint8(0) 
    |  		evtQueue(i) = event; 
    |  		paramQueue(i) = param; 
    |  		return 
    |  	end 
    |  end
  function [evtQueue, paramQueue, parameter] = BAT_Info_To_OtherRobot_dequeue(event, evtQueueIn, paramQueueIn):
    | function [evtQueue, paramQueue, parameter] = BAT_Info_To_OtherRobot_dequeue(event, evtQueueIn, paramQueueIn) %eml 
    |   evtQueue = evtQueueIn; 
    |   paramQueue = paramQueueIn; 
    |   parameter = 0; 
    |   for i = 1:length(evtQueue) 
    |     if evtQueue(i) == event 
    |          parameter = paramQueue(i); 
    |          for j = i:length(evtQueue)-1 
    |              evtQueue(j) = evtQueue(j+1); 
    |              %Compatibility 
    |              evtQueue(j+length(evtQueue)) = evtQueue(j+1+length(evtQueue)); 
    |              paramQueue(j) = paramQueue(j+1); 
    |          end 
    |          evtQueue(length(evtQueue)) = 0; 
    |          %Compatibility 
    |          evtQueue(length(evtQueue)+length(evtQueue)) = 0; 
    |          paramQueue(length(paramQueue)) = 0; 
    |          return 
    |      end 
    |   end
  function available = BAT_Info_To_OtherRobot_checkQueue(event, evtQueue):
    | function available = BAT_Info_To_OtherRobot_checkQueue(event, evtQueue) %eml 
    |  available = false; 
    |  for i = 1:length(evtQueue) 
    |      if evtQueue(i) == event 
    |          available = true;    
    |          return 
    |      end 
    |  end
  function [evtQueue, paramQueue] = BAT_Info_ToStrikeProcessing_enqueue(event, evtQueueIn, param, paramQueueIn):
    | function [evtQueue, paramQueue] = BAT_Info_ToStrikeProcessing_enqueue(event, evtQueueIn, param, paramQueueIn) %eml 
    |  evtQueue = evtQueueIn; 
    |  paramQueue = paramQueueIn; 
    |  for i = 1:length(evtQueue) 
    |  	if evtQueue(i) == uint8(0) 
    |  		evtQueue(i) = event; 
    |  		paramQueue(i) = param; 
    |  		return 
    |  	end 
    |  end
  function [evtQueue, paramQueue, parameter] = BAT_Info_ToStrikeProcessing_dequeue(event, evtQueueIn, paramQueueIn):
    | function [evtQueue, paramQueue, parameter] = BAT_Info_ToStrikeProcessing_dequeue(event, evtQueueIn, paramQueueIn) %eml 
    |   evtQueue = evtQueueIn; 
    |   paramQueue = paramQueueIn; 
    |   parameter = 0; 
    |   for i = 1:length(evtQueue) 
    |     if evtQueue(i) == event 
    |          parameter = paramQueue(i); 
    |          for j = i:length(evtQueue)-1 
    |              evtQueue(j) = evtQueue(j+1); 
    |              %Compatibility 
    |              evtQueue(j+length(evtQueue)) = evtQueue(j+1+length(evtQueue)); 
    |              paramQueue(j) = paramQueue(j+1); 
    |          end 
    |          evtQueue(length(evtQueue)) = 0; 
    |          %Compatibility 
    |          evtQueue(length(evtQueue)+length(evtQueue)) = 0; 
    |          paramQueue(length(paramQueue)) = 0; 
    |          return 
    |      end 
    |   end
  function available = BAT_Info_ToStrikeProcessing_checkQueue(event, evtQueue):
    | function available = BAT_Info_ToStrikeProcessing_checkQueue(event, evtQueue) %eml 
    |  available = false; 
    |  for i = 1:length(evtQueue) 
    |      if evtQueue(i) == event 
    |          available = true;    
    |          return 
    |      end 
    |  end
  function [evtQueue, paramQueue] = BAT_Info_From_SensorProcessing_enqueue(event, evtQueueIn, param, paramQueueIn):
    | function [evtQueue, paramQueue] = BAT_Info_From_SensorProcessing_enqueue(event, evtQueueIn, param, paramQueueIn) %eml 
    |  evtQueue = evtQueueIn; 
    |  paramQueue = paramQueueIn; 
    |  for i = 1:length(evtQueue) 
    |  	if evtQueue(i) == uint8(0) 
    |  		evtQueue(i) = event; 
    |  		paramQueue(i) = param; 
    |  		return 
    |  	end 
    |  end
  function [evtQueue, paramQueue, parameter] = BAT_Info_From_SensorProcessing_dequeue(event, evtQueueIn, paramQueueIn):
    | function [evtQueue, paramQueue, parameter] = BAT_Info_From_SensorProcessing_dequeue(event, evtQueueIn, paramQueueIn) %eml 
    |   evtQueue = evtQueueIn; 
    |   paramQueue = paramQueueIn; 
    |   parameter = 0; 
    |   for i = 1:length(evtQueue) 
    |     if evtQueue(i) == event 
    |          parameter = paramQueue(i); 
    |          for j = i:length(evtQueue)-1 
    |              evtQueue(j) = evtQueue(j+1); 
    |              %Compatibility 
    |              evtQueue(j+length(evtQueue)) = evtQueue(j+1+length(evtQueue)); 
    |              paramQueue(j) = paramQueue(j+1); 
    |          end 
    |          evtQueue(length(evtQueue)) = 0; 
    |          %Compatibility 
    |          evtQueue(length(evtQueue)+length(evtQueue)) = 0; 
    |          paramQueue(length(paramQueue)) = 0; 
    |          return 
    |      end 
    |   end
  function available = BAT_Info_From_SensorProcessing_checkQueue(event, evtQueue):
    | function available = BAT_Info_From_SensorProcessing_checkQueue(event, evtQueue) %eml 
    |  available = false; 
    |  for i = 1:length(evtQueue) 
    |      if evtQueue(i) == event 
    |          available = true;    
    |          return 
    |      end 
    |  end

== stateflow chart SensorProcessing/SensorProcessing_Statechart ==
  state chart
    state chartRegion [parallel]
      settings: executionOrder=2
      state Initial
        state Reading
          entry: c0=reset();
        state Sending
          entry: c0=reset();
        Reading -> Sending : [ballRecognized == true]
            | {[BAT_InfoWriteOut, BAT_InfoParamWriteOut] = BAT_Info_enqueue(EVT_TRANSFERBATINFO_POSX, BAT_InfoWriteOut, double(posX), BAT_InfoParamWriteOut)
            | [BAT_InfoWriteOut, BAT_InfoParamWriteOut] = BAT_Info_enqueue(EVT_TRANSFERBATINFO_POSY, BAT_InfoWriteOut, double(posY), BAT_InfoParamWriteOut)
            | [BAT_InfoWriteOut, BAT_InfoParamWriteOut] = BAT_Info_enqueue(EVT_TRANSFERBATINFO_POSZ, BAT_InfoWriteOut, double(posZ), BAT_InfoParamWriteOut)
            | [BAT_InfoWriteOut, BAT_InfoParamWriteOut] = BAT_Info_enqueue(EVT_TRANSFERBATINFO_TIMEOFARRIVAL, BAT_InfoWriteOut, double(timeOfArrival), BAT_InfoParamWriteOut)
            | [BAT_InfoWriteOut, BAT_InfoParamWriteOut] = BAT_Info_enqueue(EVT_TRANSFERBATINFO_VELOCITY, BAT_InfoWriteOut, double(velocity), BAT_InfoParamWriteOut)
            | ; }
        Sending -> Reading : [time(c0) >= 0.1]
    state DataInit [parallel]
      settings: executionOrder=1
    DataInit -> DataInit : {BAT_InfoWriteOut = BAT_InfoWriteIn;
        | BAT_InfoParamWriteOut = BAT_InfoParamWriteIn;
        | BAT_InfoReadOut = BAT_InfoReadIn;
        | BAT_InfoParamReadOut = BAT_InfoParamReadIn;
        | ; }
  (default) -> Reading
  (default) -> Initial
  (default) -> chart
  data: clock function_input double; logicalTime function_output uint32; clock function_output double; event function_input uint8; evtQueueIn function_input uint8 size=[10,2]; param function_input double; paramQueueIn function_input double size=[10]; evtQueue function_output uint8 size=[10,2]; paramQueue function_output double size=[10]; event function_input uint8; evtQueueIn function_input uint8 size=[10,2]; paramQueueIn function_input double size=[10]; evtQueue function_output uint8 size=[10,2]; paramQueue function_output double size=[10]; parameter function_output double; event function_input uint8; evtQueue function_input uint8 size=[10,2]; available function_output boolean; clockSignal input double; posX input double; posY input double; posZ input double; timeOfArrival input double; velocity input double; ballRecognized input boolean; BAT_InfoReadIn input uint8 size=[10,2]; BAT_InfoParamReadIn input double size=10; BAT_InfoWriteIn input uint8 size=[10,2]; BAT_InfoParamWriteIn input double size=10; BAT_InfoReadOut output uint8 size=[10,2]; BAT_InfoParamReadOut output double size=10; BAT_InfoWriteOut output uint8 size=[10,2]; BAT_InfoParamWriteOut output double size=10; EVT_TRANSFERBATINFO_POSX constant uint32 =6; EVT_TRANSFERBATINFO_POSY constant uint32 =7; EVT_TRANSFERBATINFO_POSZ constant uint32 =8; EVT_TRANSFERBATINFO_TIMEOFARRIVAL constant uint32 =9; EVT_TRANSFERBATINFO_VELOCITY constant uint32 =10; c0 local double =0.0
  function logicalTime = time(clock):
    | function logicalTime = time(clock) 
    | 
    |  sample = 0.001;  % the sample time of the system clock 
    | 
    |  %convert to pass units of time after last reset 
    | 
    |  logicalTime = uint32((clockSignal - clock)/sample);
  function clock = reset():
    | function clock = reset() 
    | 
    |  %set clock variable to current time 
    | 
    |  clock = clockSignal;
  function [evtQueue, paramQueue] = BAT_Info_enqueue(event, evtQueueIn, param, paramQueueIn):
    | function [evtQueue, paramQueue] = BAT_Info_enqueue(event, evtQueueIn, param, paramQueueIn) %eml 
    |  evtQueue = evtQueueIn; 
    |  paramQueue = paramQueueIn; 
    |  for i = 1:length(evtQueue) 
    |  	if evtQueue(i) == uint8(0) 
    |  		evtQueue(i) = event; 
    |  		paramQueue(i) = param; 
    |  		return 
    |  	end 
    |  end
  function [evtQueue, paramQueue, parameter] = BAT_Info_dequeue(event, evtQueueIn, paramQueueIn):
    | function [evtQueue, paramQueue, parameter] = BAT_Info_dequeue(event, evtQueueIn, paramQueueIn) %eml 
    |   evtQueue = evtQueueIn; 
    |   paramQueue = paramQueueIn; 
    |   parameter = 0; 
    |   for i = 1:length(evtQueue) 
    |     if evtQueue(i) == event 
    |          parameter = paramQueue(i); 
    |          for j = i:length(evtQueue)-1 
    |              evtQueue(j) = evtQueue(j+1); 
    |              %Compatibility 
    |              evtQueue(j+length(evtQueue)) = evtQueue(j+1+length(evtQueue)); 
    |              paramQueue(j) = paramQueue(j+1); 
    |          end 
    |          evtQueue(length(evtQueue)) = 0; 
    |          %Compatibility 
    |          evtQueue(length(evtQueue)+length(evtQueue)) = 0; 
    |          paramQueue(length(paramQueue)) = 0; 
    |          return 
    |      end 
    |   end
  function available = BAT_Info_checkQueue(event, evtQueue):
    | function available = BAT_Info_checkQueue(event, evtQueue) %eml 
    |  available = false; 
    |  for i = 1:length(evtQueue) 
    |      if evtQueue(i) == event 
    |          available = true;    
    |          return 
    |      end 
    |  end

== stateflow chart StrikeProcessing/StrikeProcessing_Statechart ==
  state chart
    state chartRegion [parallel]
      settings: executionOrder=2
      state Init
        state Receiving
        Receiving -> Receiving : [BAT_Info_checkQueue(EVT_TRANSFERBATINFO_POSX, BAT_InfoReadOut) && BAT_Info_checkQueue(EVT_TRANSFERBATINFO_POSY, BAT_InfoReadOut) && BAT_Info_checkQueue(EVT_TRANSFERBATINFO_POSZ, BAT_InfoReadOut) && BAT_Info_checkQueue(EVT_TRANSFERBATINFO_TIMEOFARRIVAL, BAT_InfoReadOut) && BAT_Info_checkQueue(EVT_TRANSFERBATINFO_VELOCITY, BAT_InfoReadOut)]
            | {[BAT_InfoReadOut, BAT_InfoParamReadOut, tmp_var_1] = BAT_Info_dequeue(EVT_TRANSFERBATINFO_POSX, BAT_InfoReadOut, BAT_InfoParamReadOut);
            | [BAT_InfoReadOut, BAT_InfoParamReadOut, tmp_var_2] = BAT_Info_dequeue(EVT_TRANSFERBATINFO_POSY, BAT_InfoReadOut, BAT_InfoParamReadOut);
            | [BAT_InfoReadOut, BAT_InfoParamReadOut, tmp_var_3] = BAT_Info_dequeue(EVT_TRANSFERBATINFO_POSZ, BAT_InfoReadOut, BAT_InfoParamReadOut);
            | [BAT_InfoReadOut, BAT_InfoParamReadOut, tmp_var_4] = BAT_Info_dequeue(EVT_TRANSFERBATINFO_TIMEOFARRIVAL, BAT_InfoReadOut, BAT_InfoParamReadOut);
            | [BAT_InfoReadOut, BAT_InfoParamReadOut, tmp_var_5] = BAT_Info_dequeue(EVT_TRANSFERBATINFO_VELOCITY, BAT_InfoReadOut, BAT_InfoParamReadOut); posX = tmp_var_1 ;  posY = tmp_var_2 ;  posZ = tmp_var_3 ;  timeOfArrival = tmp_var_4 ;  velocity = tmp_var_5 ; }
    state DataInit [parallel]
      settings: executionOrder=1
    DataInit -> DataInit : {BAT_InfoWriteOut = BAT_InfoWriteIn;
        | BAT_InfoParamWriteOut = BAT_InfoParamWriteIn;
        | BAT_InfoReadOut = BAT_InfoReadIn;
        | BAT_InfoParamReadOut = BAT_InfoParamReadIn;
        | ; }
  (default) -> Receiving
  (default) -> Init
  (default) -> chart
  data: posX local double; posY local double; posZ local double; timeOfArrival local double; velocity local double; clock function_input double; logicalTime function_output uint32; clock function_output double; event function_input uint8; evtQueueIn function_input uint8 size=[10,2]; param function_input double; paramQueueIn function_input double size=[10]; evtQueue function_output uint8 size=[10,2]; paramQueue function_output double size=[10]; event function_input uint8; evtQueueIn function_input uint8 size=[10,2]; paramQueueIn function_input double size=[10]; evtQueue function_output uint8 size=[10,2]; paramQueue function_output double size=[10]; parameter function_output double; event function_input uint8; evtQueue function_input uint8 size=[10,2]; available function_output boolean; clockSignal input double; BAT_InfoReadIn input uint8 size=[10,2]; BAT_InfoParamReadIn input double size=10; BAT_InfoWriteIn input uint8 size=[10,2]; BAT_InfoParamWriteIn input double size=10; BAT_InfoReadOut output uint8 size=[10,2]; BAT_InfoParamReadOut output double size=10; BAT_InfoWriteOut output uint8 size=[10,2]; BAT_InfoParamWriteOut output double size=10; EVT_TRANSFERBATINFO_POSX constant uint32 =6; EVT_TRANSFERBATINFO_POSY constant uint32 =7; EVT_TRANSFERBATINFO_POSZ constant uint32 =8; EVT_TRANSFERBATINFO_TIMEOFARRIVAL constant uint32 =9; EVT_TRANSFERBATINFO_VELOCITY constant uint32 =10; tmp_var_1 local double; tmp_var_2 local double; tmp_var_3 local double; tmp_var_4 local double; tmp_var_5 local double
  function logicalTime = time(clock):
    | function logicalTime = time(clock) 
    | 
    |  sample = 0.001;  % the sample time of the system clock 
    | 
    |  %convert to pass units of time after last reset 
    | 
    |  logicalTime = uint32((clockSignal - clock)/sample);
  function clock = reset():
    | function clock = reset() 
    | 
    |  %set clock variable to current time 
    | 
    |  clock = clockSignal;
  function [evtQueue, paramQueue] = BAT_Info_enqueue(event, evtQueueIn, param, paramQueueIn):
    | function [evtQueue, paramQueue] = BAT_Info_enqueue(event, evtQueueIn, param, paramQueueIn) %eml 
    |  evtQueue = evtQueueIn; 
    |  paramQueue = paramQueueIn; 
    |  for i = 1:length(evtQueue) 
    |  	if evtQueue(i) == uint8(0) 
    |  		evtQueue(i) = event; 
    |  		paramQueue(i) = param; 
    |  		return 
    |  	end 
    |  end
  function [evtQueue, paramQueue, parameter] = BAT_Info_dequeue(event, evtQueueIn, paramQueueIn):
    | function [evtQueue, paramQueue, parameter] = BAT_Info_dequeue(event, evtQueueIn, paramQueueIn) %eml 
    |   evtQueue = evtQueueIn; 
    |   paramQueue = paramQueueIn; 
    |   parameter = 0; 
    |   for i = 1:length(evtQueue) 
    |     if evtQueue(i) == event 
    |          parameter = paramQueue(i); 
    |          for j = i:length(evtQueue)-1 
    |              evtQueue(j) = evtQueue(j+1); 
    |              %Compatibility 
    |              evtQueue(j+length(evtQueue)) = evtQueue(j+1+length(evtQueue)); 
    |              paramQueue(j) = paramQueue(j+1); 
    |          end 
    |          evtQueue(length(evtQueue)) = 0; 
    |          %Compatibility 
    |          evtQueue(length(evtQueue)+length(evtQueue)) = 0; 
    |          paramQueue(length(paramQueue)) = 0; 
    |          return 
    |      end 
    |   end
  function available = BAT_Info_checkQueue(event, evtQueue):
    | function available = BAT_Info_checkQueue(event, evtQueue) %eml 
    |  available = false; 
    |  for i = 1:length(evtQueue) 
    |      if evtQueue(i) == event 
    |          available = true;    
    |          return 
    |      end 
    |  end
